simulink model "red_neuronal"  (R2023b)
settings: Solver=VariableStepAuto  StartTime=0.0  StopTime=10.0  RelTol=1e-3
libraries: neural x232
(part 11 of 11)

== system red_neuronal/Feed-Forward Neural Network/Layer 4/Delays 1 ==
  "p{4}" : Inport  PortDimensions=32  SampleTime=0.1
      mask Display: e = 0.06;c1 = [120 230 180]/255;c2 = ([120 230 180]+0)/(256+128);c3 = ([120 230 180]+128)/(256+128);patch([0 1 1 0],[0 0 1 1],c1);patch([0 1 1 1-e 1-e 0+e],[0 0 1 1-e 0+e 0+e],c2);patch([0 0 1 1-e 0+e 0+e],[0 1 1 1-e 1-e 0+e],c3);plot([0 1 1 0 0],[0 0 1 1 0]);
  mux : Mux  Inputs=1
      mask Display: e = 0.06;c1 = [120 150 230]/255;c2 = ([120 150 230]+0)/383;c3 = ([120 150 230]+128)/383;patch([0 1 1 0],[0 0 1 1],c1);patch([0 1 1 1-e 1-e 0+e],[0 0 1 1-e 0+e 0+e],c2);patch([0 0 1 1-e 0+e 0+e],[0 1 1 1-e 1-e 0+e],c3);plot([0 1 1 0 0],[0 0 1 1 0]);disp('Mux')
  "pd{4,3}" : Outport
      mask Display: e = 0.06;c1 = [120 230 180]/255;c2 = ([120 230 180]+0)/(256+128);c3 = ([120 230 180]+128)/(256+128);patch([0 1 1 0],[0 0 1 1],c1);patch([0 1 1 1-e 1-e 0+e],[0 0 1 1-e 0+e 0+e],c2);patch([0 0 1 1-e 0+e 0+e],[0 1 1 1-e 1-e 0+e],c3);plot([0 1 1 0 0],[0 0 1 1 0]);
  wires:
  "p{4}"/1 -> mux/1
  mux/1 -> "pd{4,3}"/1

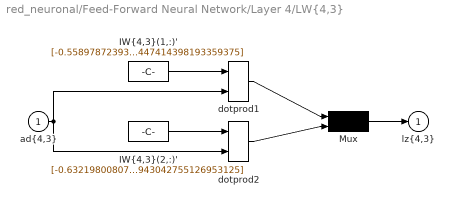
== system red_neuronal/Feed-Forward Neural Network/Layer 4/LW{4,3} ==
  "ad{4,3}" : Inport  PortDimensions=32  SampleTime=0.1
      mask Display: e = 0.06;c1 = [120 230 180]/255;c2 = ([120 230 180]+0)/(256+128);c3 = ([120 230 180]+128)/(256+128);patch([0 1 1 0],[0 0 1 1],c1);patch([0 1 1 1-e 1-e 0+e],[0 0 1 1-e 0+e 0+e],c2);patch([0 0 1 1-e 0+e 0+e],[0 1 1 1-e 1-e 0+e],c3);plot([0 1 1 0 0],[0 0 1 1 0]);
  "IW{4,3}(1,:)'" : Constant  Value=[-0.5589787239369166105262820565258152782917022705078125;-0.2070859607009855329895486875102506019175052642822265625;-0.091899834305261995925917517524794675409793853759765625;-0.10344014431906280171435952297542826272547245025634765625;-0.6596899018849951001897125024697743356227874755859375;0.60040926355066659425574471242725849151611328125;-0.7006898473202767263501300476491451263427734375;-0.76946594189258432638922613477916456758975982666015625;-0.99364088636430836221080653558601625263690948486328125;-0.067542999257727054374100816858117468655109405517578125;-0.281527839508599775353303584779496304690837860107421875;-0.086254681370532437778564371910761110484600067138671875;0.5329318444442099345081942374235950410366058349609375;-0.07736365414966679676656013953106594271957874298095703125;-0.5289925311938634688857518995064310729503631591796875;0.7686979402014733064874008050537668168544769287109375;-0.747512658413281183555909592541866004467010498046875;-0.284867825080564462947307902140892110764980316162109375;0.947739707927953478616700522252358496189117431640625;0.027225964184894112241064334511975175701081752777099609375;0.088924565843967962042171393477474339306354522705078125;-0.1401376741740854303674979064453509636223316192626953125;-0.7396344808247163893355491381953470408916473388671875;-0.3098494160749769577023471356369554996490478515625;0.704822657885754377815601401380263268947601318359375;-0.69929274907711980180380351157509721815586090087890625;0.22081730299011448348522890228196047246456146240234375;0.347869410152553626414118070897529833018779754638671875;-0.486565820635423473827785301182302646338939666748046875;0.06533032500012354859553198593857814557850360870361328125;0.55018224904682055953486496946425177156925201416015625;-0.08728694102075416905162086322889081202447414398193359375]
      mask Display: e = 0.06;c1 = [120 150 230]/255;c2 = ([120 150 230]+0)/383;c3 = ([120 150 230]+128)/383;patch([0 1 1 0],[0 0 1 1],c1);patch([0 1 1 1-e 1-e 0+e],[0 0 1 1-e 0+e 0+e],c2);patch([0 0 1 1-e 0+e 0+e],[0 1 1 1-e 1-e 0+e],c3);plot([0 1 1 0 0],[0 0 1 1 0]);disp('weights');
  "IW{4,3}(2,:)'" : Constant  Value=[-0.6321980080726825601544760502292774617671966552734375;0.2431014554436619068411573607590980827808380126953125;0.10172730120339502912774065634948783554136753082275390625;-0.78659638198894887839429657105938531458377838134765625;0.293425221996985730044116280623711645603179931640625;0.1388499546431294362491826177574694156646728515625;0.95202522533518585401424161318573169410228729248046875;0.787723639246415086034858177299611270427703857421875;0.341009942634940443895175121724605560302734375;-0.85246297979437957170745221446850337088108062744140625;0.5646642049490953052526265310007147490978240966796875;-0.0980243208539182120375699014402925968170166015625;-0.6029639883735578020917955655022524297237396240234375;0.45505435028109919581851272596395574510097503662109375;0.62768276242448373114513060500030405819416046142578125;0.58150004570820768012850976447225548326969146728515625;0.5408064758967168206282849496346898376941680908203125;0.06036640136897201969201631754913250915706157684326171875;0.1815009512243725697810958763511735014617443084716796875;-0.01455741576356261481051124206942404271103441715240478515625;0.82862025659562632551313754447619430720806121826171875;0.74850609377396704058327259190264157950878143310546875;0.8494822094771226073106618059682659804821014404296875;0.326212414650591642217847265783348120748996734619140625;-0.6852477750865337835506352348602376878261566162109375;-0.134027168318218981024614322450361214578151702880859375;-0.5490241184861972545405706114252097904682159423828125;-0.52818380359787087119372017696150578558444976806640625;0.91385942535486830440305539013934321701526641845703125;0.7781343938318772135431800052174367010593414306640625;-0.0511751785544490578327980756512260995805263519287109375;-0.80325171305120879328143246311810798943042755126953125]
      mask Display: e = 0.06;c1 = [120 150 230]/255;c2 = ([120 150 230]+0)/383;c3 = ([120 150 230]+128)/383;patch([0 1 1 0],[0 0 1 1],c1);patch([0 1 1 1-e 1-e 0+e],[0 0 1 1-e 0+e 0+e],c2);patch([0 0 1 1-e 0+e 0+e],[0 1 1 1-e 1-e 0+e],c3);plot([0 1 1 0 0],[0 0 1 1 0]);disp('weights');
  Mux : Mux  Inputs=2
      mask Display: e = 0.06;c1 = [120 150 230]/255;c2 = ([120 150 230]+0)/383;c3 = ([120 150 230]+128)/383;patch([0 1 1 0],[0 0 1 1],c1);patch([0 1 1 1-e 1-e 0+e],[0 0 1 1-e 0+e 0+e],c2);patch([0 0 1 1-e 0+e 0+e],[0 1 1 1-e 1-e 0+e],c3);plot([0 1 1 0 0],[0 0 1 1 0]);disp('Mux');
  dotprod1 : neural/Weight Functions/dotprod
  dotprod2 : neural/Weight Functions/dotprod
  "lz{4,3}" : Outport
      mask Display: e = 0.06;c1 = [120 230 180]/255;c2 = ([120 230 180]+0)/(256+128);c3 = ([120 230 180]+128)/(256+128);patch([0 1 1 0],[0 0 1 1],c1);patch([0 1 1 1-e 1-e 0+e],[0 0 1 1-e 0+e 0+e],c2);patch([0 0 1 1-e 0+e 0+e],[0 1 1 1-e 1-e 0+e],c3);plot([0 1 1 0 0],[0 0 1 1 0]);
  wires:
  "IW{4,3}(1,:)'"/1 -> dotprod1/1
  "ad{4,3}"/1 -> dotprod1/2, dotprod2/2
  dotprod1/1 -> Mux/1
  "IW{4,3}(2,:)'"/1 -> dotprod2/1
  dotprod2/1 -> Mux/2
  Mux/1 -> "lz{4,3}"/1
